simulink model "UAV_PIL"  (Simulink 7.5)
settings: Solver=ode3  StartTime=0.0  StopTime=inf  FixedStep=SampleTime  RelTol=1e-3
values from neighbouring files (symbols this model uses):
  SampleTime = 0.02    [setup.m]
  TimeDelay = 0.00    (= 0)    [setup.m]
undefined symbols (not defined in the file or in its folder): Serial_Port, Standard_Devices
libraries: simulink_extras x14, simulink x7, Actuator_Lib x2, etargetslib x2, rtwinlib x2, aerolibfltsims x2, NonlinearModel_Lib x1, Sensors_Lib x1
CloseFcn:
  | rtwprivate ssgencode ModelCloseRequest Good_NL_model
settings Model: Creator=Paul  LastModifiedBy=dept of AEM  SimulationMode=external  ExtModeTrigDuration=100000
settings DataIOCC: TimeSaveName=time
settings OptimizationCC: InitFltsAndDblsToZero=on
settings DebuggingCC: StrictBusMsg=Warning
settings HardwareCC: ProdIntDivRoundTo=Zero  ProdEndianess=LittleEndian  ProdHWDeviceType=Generic->32-bit x86 compatible
settings RTWCC: SystemTargetFile=rtwin.tlc  TemplateMakefile=rtwin.tmf  Description=Real-Time Windows Target  ProcessScript=rtwin_make_rtw_hook  RTWCompilerOptimization=On
settings CodeAppCC: MaxIdLength=95
settings RTWinTargetCC: TargetLibSuffix=_rtwin.lib  TargetPreCompLibLocation=C:\Program Files\MATLAB\R2010a\toolbox\rtw\targets\rtwin\lib  TargetFunctionLibrary=ANSI_C  ERTCodeCoverageTool=None  PortableWordSizes=off

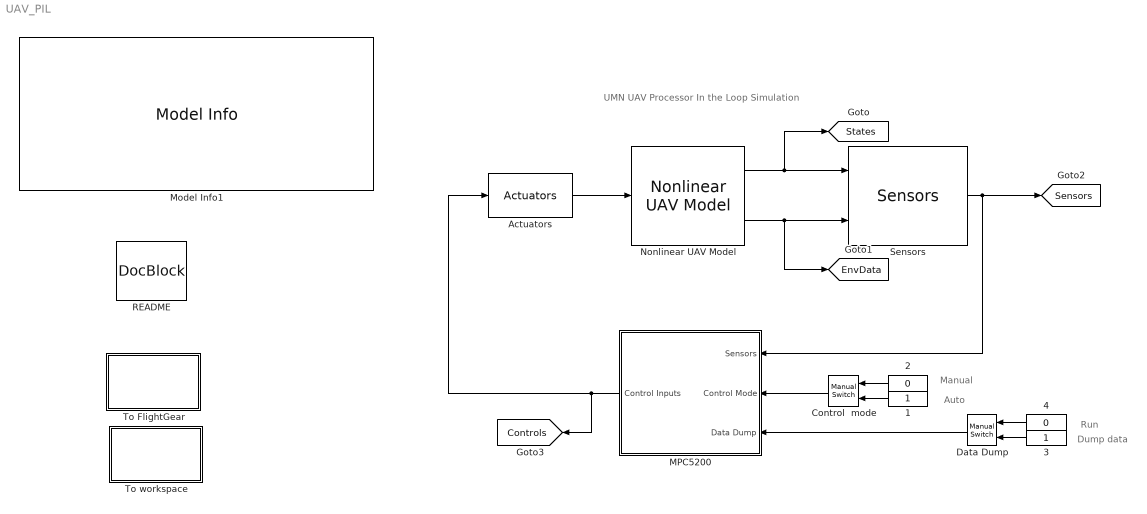
== system UAV_PIL ==
  note: Manual
  note: Auto
  note: UMN UAV
      | Processor In the Loop Simulation
  note: Run
  note: Dump data
  1 : Constant  OutDataTypeMode=uint8  OutDataType=sfix(16)  OutScaling=2^0  OutDataTypeStr=uint8
  2 : Constant  Value=0  OutDataTypeMode=uint8  OutDataType=sfix(16)  OutScaling=2^0  OutDataTypeStr=uint8
  3 : Constant  OutDataTypeMode=uint8  OutDataType=sfix(16)  OutScaling=2^0  OutDataTypeStr=uint8
  4 : Constant  Value=0  OutDataTypeMode=uint8  OutDataType=sfix(16)  OutScaling=2^0  OutDataTypeStr=uint8
  Actuators : Actuator_Lib/Actuators  SystemSampleTime=-1
  Control  mode : simulink/Signal Routing/Manual Switch  SystemSampleTime=-1  sw=1  action=0  varsize=off
  Data Dump : simulink/Signal Routing/Manual Switch  SystemSampleTime=-1  sw=1  action=0  varsize=off
  MPC5200 : Subsystem
  Model Info1 : simulink/Model-Wide Utilities/Model Info  SystemSampleTime=-1  InitialBlockCM=None  BlockCM=None  Frame=on  DisplayStringWithTags=|  HorizontalTextAlignment=Left  LeftAlignmentValue=0.02  SourceBlockDiagram=UAV_PIL  TagMaxNumber=20
      | MODEL INFORMATION
      | UMN UAV Processor-in-the-Loop Simulation
      | 
      | University of Minnesota
      | Aerospace Engineering and Mechanics
      | Copyright 2011 Regents of the University of Minnesota. All rights reserved.
      | 
      | == SVN Info ==
      | %<ModelVersion>
      | Last modified by %<LastModifiedBy> on %<LastModificationDate>
  Nonlinear UAV Model : NonlinearModel_Lib/Nonlinear UAV Model  SystemSampleTime=-1
  README : simulink/Model-Wide Utilities/DocBlock  SystemSampleTime=-1  DocumentType=Text
  Sensors : Sensors_Lib/Sensors  SystemSampleTime=-1
  To FlightGear : Subsystem
      mask Display: text(0.1,.5, 'To FlightGear')
  To workspace : Subsystem
      mask Display: text(0.1,.5, 'To Workspace')
  tag scope: Controls=global, EnvData=global, Sensors=global, States=global
  wires:
  Nonlinear UAV Model/1 -> Sensors/1, [States]
  Nonlinear UAV Model/2 -> Sensors/2, [EnvData]
  Actuators/1 -> Nonlinear UAV Model/1
  2/1 -> Control  mode/1
  1/1 -> Control  mode/2
  Control  mode/1 -> MPC5200/2(Control Mode)
  MPC5200/1(Control Inputs) -> [Controls], Actuators/1
  Sensors/1 -> MPC5200/1(Sensors), [Sensors]
  4/1 -> Data Dump/1
  3/1 -> Data Dump/2
  Data Dump/1 -> MPC5200/3(Data Dump)

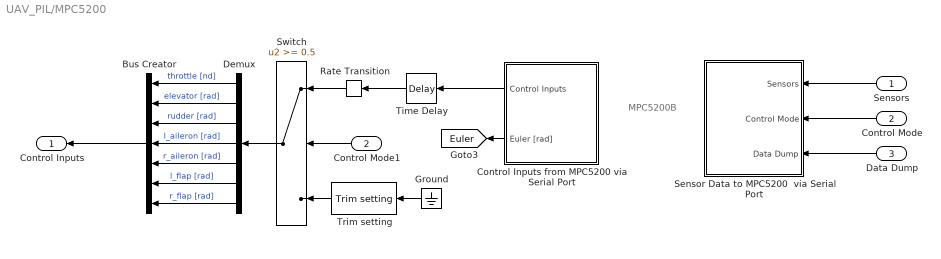
== system UAV_PIL/MPC5200 ==
  note: MPC5200B
  Sensors : Inport
  Control Mode : Inport  Port=2
  Data Dump : Inport  Port=3
  Bus Creator : BusCreator  Inputs=7
  Control Inputs from MPC5200 via Serial Port : Subsystem
  Control Mode1 : InportShadow  Port=2
  Demux : Demux  Outputs=7
  Ground : Ground
  Rate Transition : RateTransition
  Sensor Data to MPC5200  via Serial Port : Subsystem
  Switch : Switch  Threshold=0.5  OutDataType=fixdt(1, 16)  OutScaling=2^0
  Time Delay : TransportDelay  DelayTime=TimeDelay  FixedBuffer=on
  "Trim setting " : Actuator_Lib/Trim setting   SystemSampleTime=-1
  Control Inputs : Outport  OutDataType=sfix(16)  OutScaling=2^0
  tag scope: Euler=global
  wires:
  Control Inputs from MPC5200 via Serial Port/1(Control Inputs) -> Time Delay/1
  Ground/1 -> "Trim setting "/1
  "Trim setting "/1 -> Switch/3
  Rate Transition/1 -> Switch/1
  Time Delay/1 -> Rate Transition/1
  Control Mode/1 -> Sensor Data to MPC5200  via Serial Port/2(Control Mode)
  Control Mode1/1 -> Switch/2
  Demux/1 -> Bus Creator/1  "throttle [nd]"
  Demux/2 -> Bus Creator/2  "elevator [rad]"
  Demux/3 -> Bus Creator/3  "rudder [rad]"
  Demux/4 -> Bus Creator/4  "l_aileron [rad]"
  Demux/5 -> Bus Creator/5  "r_aileron [rad]"
  Demux/6 -> Bus Creator/6  "l_flap [rad]"
  Demux/7 -> Bus Creator/7  "r_flap [rad]"
  Bus Creator/1 -> Control Inputs/1
  Switch/1 -> Demux/1
  Sensors/1 -> Sensor Data to MPC5200  via Serial Port/1(Sensors)
  Control Inputs from MPC5200 via Serial Port/2(Euler [rad]) -> [Euler]
  Data Dump/1 -> Sensor Data to MPC5200  via Serial Port/3(Data Dump)

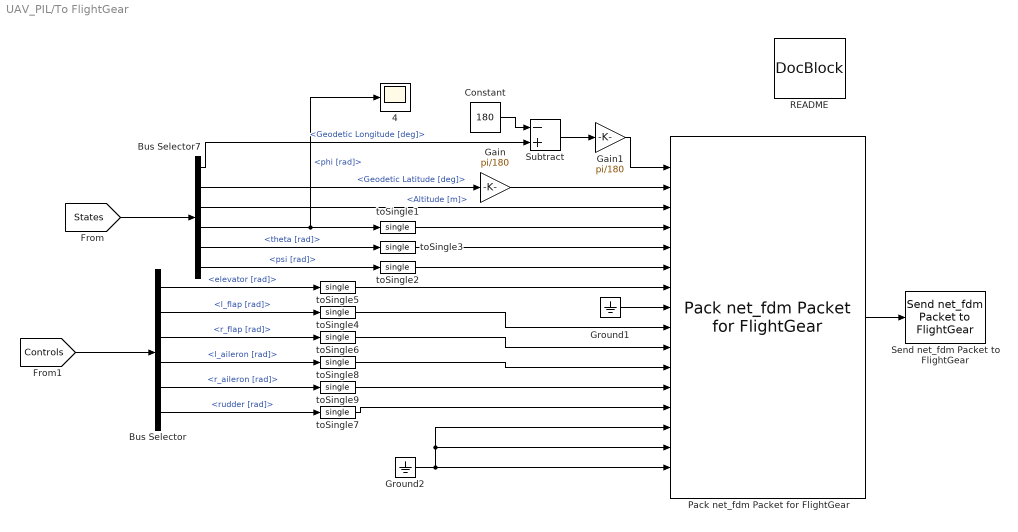
== system UAV_PIL/To FlightGear ==
  4 : Scope
      settings: TimeRange=10  YMin=-0.4  YMax=0.5  SaveName=ScopeData8
  Bus Selector : BusSelector  OutputSignals=elevator [rad],l_flap [rad],r_flap [rad],l_aileron [rad],r_aileron [rad],rudder [rad]
  Bus Selector7 : BusSelector  OutputSignals=Nav.Geodetic Longitude [deg],Nav.Geodetic Latitude [deg],Nav.Altitude [m],Euler [rad].phi [rad],Euler [rad].theta [rad],Euler [rad].psi [rad]
  Constant : Constant  Value=180  OutDataType=fixdt(1, 16)  OutScaling=2^0
  Gain : Gain  Gain=pi/180  ParameterDataType=fixdt(1, 16)  ParameterScaling=2^0  OutDataType=fixdt(1, 16)  OutScaling=2^0
  Gain1 : Gain  Gain=pi/180  ParameterDataType=fixdt(1, 16)  ParameterScaling=2^0  OutDataType=fixdt(1, 16)  OutScaling=2^0
  Ground1 : Ground
  Ground2 : Ground
  Pack net_fdm Packet for FlightGear : aerolibfltsims/Pack net_fdm Packet for FlightGear  FlightGearVersion=v1.9.1  ShowPositionAttitudeInputs=on  ShowVelocityAccelerationInputs=off  ShowControlSurfacePositionInputs=on  ShowEngineFuelInputs=off  ShowLandingGearInputs=off  ShowEnvironmentInputs=off  SampleTime=-1
  README : simulink/Model-Wide Utilities/DocBlock  SystemSampleTime=-1  DocumentType=Text
  Send net_fdm Packet to FlightGear : aerolibfltsims/Send net_fdm Packet to FlightGear  DestinationIpAddress=127.0.0.1  DestinationPort=5500  LocalIpPort=-1  varLen=off  SampleTime=-1
  Subtract : Sum  Inputs=-+  OutDataType=fixdt(1, 16)  OutScaling=2^-10
  toSingle{1..9} (9 alike) : DataTypeConversion  OutDataTypeMode=single  OutDataType=sfix(16)  OutScaling=2^0  OutDataTypeStr=single
  wires:
  Pack net_fdm Packet for FlightGear/1 -> Send net_fdm Packet to FlightGear/1
  Ground1/1 -> Pack net_fdm Packet for FlightGear/8
  toSingle5/1 -> Pack net_fdm Packet for FlightGear/7
  toSingle7/1 -> Pack net_fdm Packet for FlightGear/13
  Bus Selector/1 -> toSingle5/1  "<elevator [rad]>"
  Bus Selector/3 -> toSingle6/1  "<r_flap [rad]>"
  Bus Selector/6 -> toSingle7/1  "<rudder [rad]>"
  Ground2/1 -> Pack net_fdm Packet for FlightGear/16, Pack net_fdm Packet for FlightGear/15, Pack net_fdm Packet for FlightGear/14
  toSingle2/1 -> Pack net_fdm Packet for FlightGear/6
  toSingle3/1 -> Pack net_fdm Packet for FlightGear/5
  toSingle1/1 -> Pack net_fdm Packet for FlightGear/4
  [States] -> Bus Selector7/1
  [Controls] -> Bus Selector/1
  Bus Selector7/4 -> toSingle1/1, 4/1  "<phi [rad]>"
  Bus Selector7/5 -> toSingle3/1  "<theta [rad]>"
  Bus Selector7/6 -> toSingle2/1  "<psi [rad]>"
  Bus Selector7/2 -> Gain/1  "<Geodetic Latitude [deg]>"
  Bus Selector7/3 -> Pack net_fdm Packet for FlightGear/3  "<Altitude [m]>"
  Gain/1 -> Pack net_fdm Packet for FlightGear/2
  Subtract/1 -> Gain1/1
  Constant/1 -> Subtract/1
  Gain1/1 -> Pack net_fdm Packet for FlightGear/1
  Bus Selector7/1 -> Subtract/2  "<Geodetic Longitude [deg]>"
  Bus Selector/2 -> toSingle4/1  "<l_flap [rad]>"
  toSingle4/1 -> Pack net_fdm Packet for FlightGear/9
  toSingle6/1 -> Pack net_fdm Packet for FlightGear/10
  Bus Selector/4 -> toSingle8/1  "<l_aileron [rad]>"
  toSingle8/1 -> Pack net_fdm Packet for FlightGear/11
  toSingle9/1 -> Pack net_fdm Packet for FlightGear/12
  Bus Selector/5 -> toSingle9/1  "<r_aileron [rad]>"

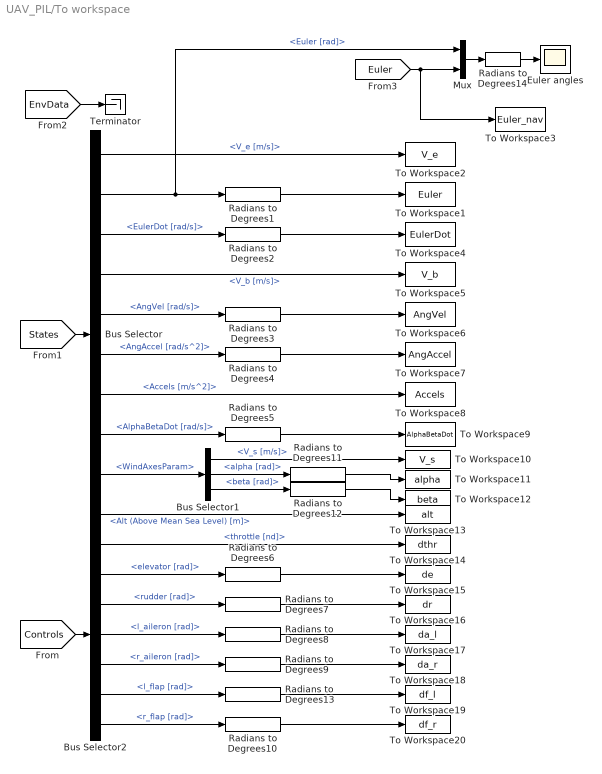
== system UAV_PIL/To workspace ==
  Bus Selector : BusSelector  OutputSignals=V_e [m/s],Euler [rad],EulerDot [rad/s],V_b [m/s],AngVel [rad/s],AngAccel [rad/s^2],Accels [m/s^2],AlphaBetaDot [rad/s],WindAxesParam,Nav.Alt (Above Mean Sea Level) [m]
  Bus Selector1 : BusSelector  OutputSignals=V_s [m/s],alpha [rad],beta [rad]
  Bus Selector2 : BusSelector  OutputSignals=throttle [nd],elevator [rad],rudder [rad],l_aileron [rad],r_aileron [rad],l_flap [rad],r_flap [rad]
  Euler angles : Scope
      settings: TimeRange=10  YMin=-40  YMax=140
  Mux : Mux  Inputs=2
  Radians to Degrees{1..14} (14 alike) : simulink_extras/Transformations/Radians to Degrees  SystemSampleTime=-1
  Terminator : Terminator
  To Workspace1 : ToWorkspace  VariableName=Euler  SampleTime=-1  SaveFormat=Array
  To Workspace10 : ToWorkspace  VariableName=V_s  SampleTime=-1  SaveFormat=Array
  To Workspace11 : ToWorkspace  VariableName=alpha  SampleTime=-1  SaveFormat=Array
  To Workspace12 : ToWorkspace  VariableName=beta  SampleTime=-1  SaveFormat=Array
  To Workspace13 : ToWorkspace  VariableName=alt  SampleTime=-1  SaveFormat=Array
  To Workspace14 : ToWorkspace  VariableName=dthr  SampleTime=-1  SaveFormat=Array
  To Workspace15 : ToWorkspace  VariableName=de  SampleTime=-1  SaveFormat=Array
  To Workspace16 : ToWorkspace  VariableName=dr  SampleTime=-1  SaveFormat=Array
  To Workspace17 : ToWorkspace  VariableName=da_l  SampleTime=-1  SaveFormat=Array
  To Workspace18 : ToWorkspace  VariableName=da_r  SampleTime=-1  SaveFormat=Array
  To Workspace19 : ToWorkspace  VariableName=df_l  SampleTime=-1  SaveFormat=Array
  To Workspace2 : ToWorkspace  VariableName=V_e  SampleTime=-1  SaveFormat=Array
  To Workspace20 : ToWorkspace  VariableName=df_r  SampleTime=-1  SaveFormat=Array
  To Workspace3 : ToWorkspace  VariableName=Euler_nav  SampleTime=-1  SaveFormat=Array
  To Workspace4 : ToWorkspace  VariableName=EulerDot  SampleTime=-1  SaveFormat=Array
  To Workspace5 : ToWorkspace  VariableName=V_b  SampleTime=-1  SaveFormat=Array
  To Workspace6 : ToWorkspace  VariableName=AngVel  SampleTime=-1  SaveFormat=Array
  To Workspace7 : ToWorkspace  VariableName=AngAccel  SampleTime=-1  SaveFormat=Array
  To Workspace8 : ToWorkspace  VariableName=Accels  SampleTime=-1  SaveFormat=Array
  To Workspace9 : ToWorkspace  VariableName=AlphaBetaDot  SampleTime=-1  SaveFormat=Array
  wires:
  Bus Selector/1 -> To Workspace2/1  "<V_e [m/s]>"
  Bus Selector/2 -> Radians to Degrees1/1, Mux/1  "<Euler [rad]>"
  Bus Selector/3 -> Radians to Degrees2/1  "<EulerDot [rad/s]>"
  Bus Selector/4 -> To Workspace5/1  "<V_b [m/s]>"
  Bus Selector/5 -> Radians to Degrees3/1  "<AngVel [rad/s]>"
  Bus Selector/6 -> Radians to Degrees4/1  "<AngAccel [rad/s^2]>"
  Bus Selector/7 -> To Workspace8/1  "<Accels [m/s^2]>"
  Bus Selector/8 -> Radians to Degrees5/1  "<AlphaBetaDot [rad/s]>"
  Bus Selector/10 -> To Workspace13/1  "<Alt (Above Mean Sea Level) [m]>"
  Radians to Degrees1/1 -> To Workspace1/1
  Radians to Degrees2/1 -> To Workspace4/1
  Radians to Degrees3/1 -> To Workspace6/1
  Radians to Degrees4/1 -> To Workspace7/1
  Radians to Degrees5/1 -> To Workspace9/1
  Bus Selector/9 -> Bus Selector1/1  "<WindAxesParam>"
  Bus Selector1/1 -> To Workspace10/1  "<V_s [m/s]>"
  Bus Selector1/2 -> Radians to Degrees11/1  "<alpha [rad]>"
  Bus Selector1/3 -> Radians to Degrees12/1  "<beta [rad]>"
  Radians to Degrees11/1 -> To Workspace11/1
  Radians to Degrees12/1 -> To Workspace12/1
  Bus Selector2/1 -> To Workspace14/1  "<throttle [nd]>"
  Bus Selector2/2 -> Radians to Degrees6/1  "<elevator [rad]>"
  Bus Selector2/3 -> Radians to Degrees7/1  "<rudder [rad]>"
  Bus Selector2/4 -> Radians to Degrees8/1  "<l_aileron [rad]>"
  Bus Selector2/5 -> Radians to Degrees9/1  "<r_aileron [rad]>"
  Bus Selector2/6 -> Radians to Degrees13/1  "<l_flap [rad]>"
  Bus Selector2/7 -> Radians to Degrees10/1  "<r_flap [rad]>"
  Radians to Degrees6/1 -> To Workspace15/1
  [Controls] -> Bus Selector2/1
  [States] -> Bus Selector/1
  [EnvData] -> Terminator/1
  [Euler] -> Mux/2, To Workspace3/1
  Mux/1 -> Radians to Degrees14/1
  Radians to Degrees14/1 -> Euler angles/1
  Radians to Degrees7/1 -> To Workspace16/1
  Radians to Degrees8/1 -> To Workspace17/1
  Radians to Degrees9/1 -> To Workspace18/1
  Radians to Degrees13/1 -> To Workspace19/1
  Radians to Degrees10/1 -> To Workspace20/1

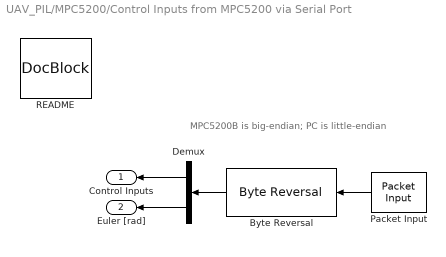
== system UAV_PIL/MPC5200/Control Inputs from MPC5200 via Serial Port ==
  note: MPC5200B is big-endian;
      | PC is little-endian
  Byte Reversal : etargetslib/Byte Reversal  numInp=1
  Demux : Demux  Outputs=[7 3]
  Packet Input : rtwinlib/Packet Input  SampleTime=SampleTime  DrvName=Standard_Devices/Serial_Port  DrvAddress=2  DrvOptions=[115200 8 0 0 0 0 0]  PacketSize=80  DataTypes='10*double'  ShowReady=off  ShowError=off  PacketID=1  ShowTimestamp=off
      settings: AttributesFormatString=Standard Devices\nSerial Port [2h]
  README : simulink/Model-Wide Utilities/DocBlock  SystemSampleTime=-1  DocumentType=Text
      content=|
      | Control Inputs
      |
      | This block contains the serial interface to the MPC5200B that recieves the
      | actuator commands. The commands are in the following order, and are sent
      | as double precision (8 bytes each). Units are radians.
      |
      | Throttle (0-1)
      | Elevator
      | Rudder
      | Left Aileron
      | Right Aileron
      | Left Flap
      | Right Flap
  Control Inputs : Outport  OutDataType=sfix(16)  OutScaling=2^0
  Euler [rad] : Outport  Port=2  OutDataType=sfix(16)  OutScaling=2^0
  wires:
  Packet Input/1 -> Byte Reversal/1
  Byte Reversal/1 -> Demux/1
  Demux/1 -> Control Inputs/1
  Demux/2 -> Euler [rad]/1

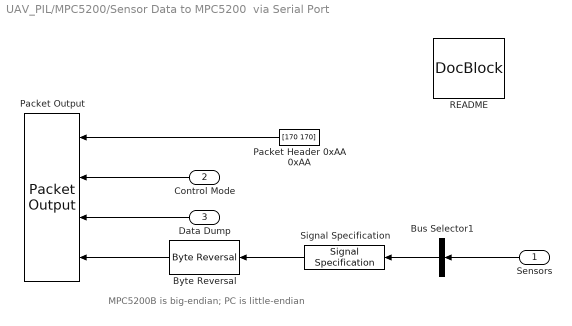
== system UAV_PIL/MPC5200/Sensor Data to MPC5200  via Serial Port ==
  note: MPC5200B is big-endian;
      | PC is little-endian
  Sensors : Inport
  Control Mode : Inport  Port=2
  Data Dump : Inport  Port=3
  Bus Selector1 : BusSelector  OutputSignals=p [rad/s],q [rad/s],r [rad/s],Ax [m/s^2],Ay [m/s^2],Az [m/s^2],Magnetic Field [nT],Geodetic Latitude [deg],Geodetic Longitude [deg],Altitude [m],Xdot [m/s],Ydot [m/s],Zdot [m/s],alpha [rad],beta [rad],Pd [Kpa],Ps [Kpa]  OutputAsBus=on
  Byte Reversal : etargetslib/Byte Reversal  numInp=1
  Packet Header 0xAA 0xAA : Constant  Value=[170 170]  OutDataTypeMode=uint8  OutDataType=sfix(16)  OutScaling=2^0  OutDataTypeStr=uint8
  Packet Output : rtwinlib/Packet Output  SampleTime=SampleTime  DrvName=Standard_Devices/Serial_Port  DrvAddress=2  DrvOptions=[115200 8 0 0 0 0 0]  PacketSize=156  DataTypes={'2*uint8','uint8','uint8','19*double'}  ShowReady=off  ShowError=off  PacketID=1  InitialValue=[]  FinalValue=[]
      settings: AttributesFormatString=Standard Devices\nSerial Port [2h]
  README : simulink/Model-Wide Utilities/DocBlock  SystemSampleTime=-1  DocumentType=Text
  Signal Specification : SignalSpecification  Dimensions=19  DataType=double  OutDataType=fixdt(1, 16)  OutScaling=2^0  OutDataTypeStr=double
  wires:
  Sensors/1 -> Bus Selector1/1
  Packet Header 0xAA 0xAA/1 -> Packet Output/1
  Byte Reversal/1 -> Packet Output/4
  Control Mode/1 -> Packet Output/2
  Signal Specification/1 -> Byte Reversal/1
  Data Dump/1 -> Packet Output/3
  Bus Selector1/1 -> Signal Specification/1
